simulink model "benchmark_model_2"  (R2021a)
settings: Solver=ode1  StartTime=0.0  StopTime=Tend  FixedStep=0.0001  MaxStep=0.1  MinStep=0.0001  AbsTol=0.01  EnableMultiTasking=on
values from neighbouring files (symbols this model uses):
  A1 = 0.00017774967488    [engine_data.mat]
  A2 = 740220.330082    [engine_data.mat]
  AL = [6 6.5 7 7.5 8 8.5 9 9.5 10 10.5 11 11.5 ... (33 elements, 33x1)]    [engine_data.mat]
  AM0 = 0.02884    [engine_data.mat]
  AREA = 0.00580880481649    [engine_data.mat]
  BORE = 0.086    [engine_data.mat]
  C_EGR = 1.5    [engine_data.mat]
  c_f = 800000    [engine_data.mat]
  c_T = 1    [engine_data.mat]
  CAIR = [0 0 0 0.21 0 0 0.79]    [engine_data.mat]
  cCO = 0    [engine_data.mat]
  cCO2 = 0    [engine_data.mat]
  cH2 = 0    [engine_data.mat]
  cH2O = 0    [engine_data.mat]
  cHC = 0    [engine_data.mat]
  cN2 = 0.79    [engine_data.mat]
  CO = [22.3416398376 20.8398063107 19.3759939408 17.9445472871 16.538827802 15.1528221174 13.7819470707 12.4234138404 11.076283262 9.74128071245 8.42044156849 7.11667724438 ... (33 elements, 33x1)]    [engine_data.mat]
  CO2 = [1.08016197936 1.63070203699 2.20578946805 2.80905596198 3.44329822989 4.11013545224 4.80975559522 5.54078746844 6.30033629562 7.08419123341 7.88717005398 8.70352822078 ... (33 elements, 33x1)]    [engine_data.mat]
  cO2 = 0.21    [engine_data.mat]
  DEN0 = 1.17881164668    [engine_data.mat]
  EGR_dia = 0.02    [engine_data.mat]
  EGR_sk = 0.125663706144    [engine_data.mat]
  EX_AREA = 0.00137444678595    [engine_data.mat]
  EX_M_AR = 0.0258532162804    [engine_data.mat]
  EXO = 40    [engine_data.mat]
  FD0 = 5    [engine_data.mat]
  FOM = [12 11.348 6.233 5 5.449 8.523 5]    [engine_data.mat]
  FR0 = 0    [engine_data.mat]
  FR_C1 = 305.731    [engine_data.mat]
  FR_C2 = 1.70183    [engine_data.mat]
  FR_C3 = 3188.7424    [engine_data.mat]
  FR_C4 = 0.000296028194151    [engine_data.mat]
  FR_C5 = 1.03    [engine_data.mat]
  H2 = [17.3855302766 15.0102176452 12.8820660449 10.9850020715 9.30240027035 7.81790027685 6.51548255669 5.37933989743 4.39378660966 3.5433012035 2.8127075229 2.1874445405 ... (33 elements, 33x1)]    [engine_data.mat]
  H2O = [3.81120036781 5.32559240945 6.64944794012 7.79700886885 8.78142378855 9.61507632366 10.310008356 10.8782622871 11.3320540899 11.6837509075 11.9456809954 12.1298414055 ... (33 elements, 33x1)]    [engine_data.mat]
  HC = [5481.3024964 4476.06435729 3754.34247414 3215.30411383 2799.83726136 2471.30975971 2205.97110777 1987.83348465 1805.78690133 1651.89669698 1520.35918152 1406.8402103 ... (33 elements, 33x1)]    [engine_data.mat]
  INC = 0    [engine_data.mat]
  INO = -40    [engine_data.mat]
  KET = 0.001    [engine_data.mat]
  Kex = 1.28224854645    [engine_data.mat]
  Kh = 0.00462    [engine_data.mat]
  MAS0 = 0.00471524658673    [engine_data.mat]
  MCh = 0.000588883862304    [engine_data.mat]
  MHC = 0.01383448    [engine_data.mat]
  MN2 = 0.028    [engine_data.mat]
  MO2 = 0.032    [engine_data.mat]
  MOLcylT = 0.00157069204711    [engine_data.mat]
  N2 = [54.5020363032 56.4529864816 58.2465252261 59.8999246568 61.4284172656 62.8453054261 64.1621746691 65.3891205654 66.5349581592 67.6074047194 68.6132342687 69.5584035698 ... (33 elements, 33x1)]    [engine_data.mat]
  O2 = [0.331300985803 0.293088680307 0.264743132617 0.242930742419 0.225648917415 0.211629427842 0.200034641439 0.190292592782 0.182002893523 0.174881554044 0.168729672297 0.163420998081 ... (33 elements, 33x1)]    [engine_data.mat]
  PR0 = 101324.72    [engine_data.mat]
  R150 = 157.079632679    [engine_data.mat]
  Rabs = 8.31441    [engine_data.mat]
  SPEC = [4 0.086 0.086 0.043 0.14665 14 1 0.1 0 0.5 0.005 0 ... (19 elements, 19x1)]    [engine_data.mat]
  TBORE = 0.055    [engine_data.mat]
  Tend = 120    [engine_data.mat]
  Th_HC = 0.1    [engine_data.mat]
  Th_knock = 0.401961937891    [engine_data.mat]
  THEX = [0 1 2 3 4 5 6 7 8 9 10 11 ... (721 elements, 1x721)]    [engine_data.mat]
  THIN = [0 1 2 3 4 5 6 7 8 9 10 11 ... (721 elements, 1x721)]    [engine_data.mat]
  TM0 = 298.15    [engine_data.mat]
  Tstart = 5    [engine_data.mat]
  TW0 = 353.15    [engine_data.mat]
  V_EX = 0.0001    [engine_data.mat]
  VAREX = [0 0 0 0 0 0 0 0 0 0 0 0 ... (721 elements, 1x721)]    [engine_data.mat]
  VARIN = [0 0 0 0 0 0 0 0 0 0 0 0 ... (721 elements, 1x721)]    [engine_data.mat]
  VH = 0.000499557214218    [engine_data.mat]
  VT = 3.84274780168e-05    [engine_data.mat]
  WOM = [0.01383448 0.04401 0.02801 0.032 0.002016 0.018016 0.028]    [engine_data.mat]
  y = 1.81    [engine_data.mat]
undefined symbols (not defined in the file or in its folder): DiscIntNeverNeededParam
libraries: pid_lib x3
(part 7 of 7)

== matlab function benchmark_model_2/ENGINE/engine_s/cylinders/cyl2/cyl/frame/ratio_burnt1/murnt_ratio/Embedded MATLAB Function ==
  data: u input; q output; Web input; Q output
function [q,Q]  = func_webC_s(u,Web)
% made by Alex on January 28th, 2010
%   y: burnt ratio
%   u: crank angle that takes 0 at the compression TDC
% Web: parameters
%
WebA = Web(1);
WebM = Web(2);
WebT = Web(3);
WebS = Web(4);
WWebs = pi-WebS;

uu = mod(u,4*pi)-WWebs;
if (uu>0)   
    q = 1.0/WebT*(WebM+1.0)*WebA*(uu/WebT)^WebM*...
          exp(-WebA*(uu/WebT)^(WebM+1.0));
    Q = 1-exp(-WebA*(uu/WebT)^(WebM+1.0));
else
    q = 0;
    Q = 0;
end

== matlab function benchmark_model_2/ENGINE/engine_s/ex_chamber/cal_flow ==
  data: area input; fen output; inlet input; c_in input; outlet input; c_out input; fml output; WOM input
function [fen,fml] = func_nozzle(area,inlet,c_in,outlet,c_out,WOM) 
% made by Alex on February 3rd, 2010
% This program calculates the flow rate through the nozzle 
% under the assamption that the mass, the energy and the mometum
% are conserved between the inlet and the outlet flows.
%
% The inlet and the outlet are connected with the sign convention 
% of the calculated flow. The sign of the flow from th einlet and 
% the outlet is positive.
%
% inlet(1):pressure 
% inlet(2):density
% inlet(3):weight of molecule
% inlet(4):degree of freedom
% outlet(1):pressure 
% outlet(2):density
% outlet(3):weight of molecule
% outlet(4):degree of freedom

y = zeros(8,1); % modified 

du = inlet(1);
if du<0
    du=0;
end
pu = inlet(2);
mu = inlet(3);
fu = inlet(4);
dd = outlet(1);
pd = outlet(2);
md = outlet(3);
fd = outlet(4);
AR = area;

if (pu >= pd)
    rp = pd/pu;
    k = (fu + 2.0)/fu;
    crp = 1.0/(k + 1.0);
    A = AR*sqrt((k + 1.0)/(2.0*k)*pu*du);
    B = sqrt((k/(k + 1.0))^2 - (0.99 - 1.0/(k + 1.0))^2);
    C = -(0.99 - 1.0/(k + 1.0))/B;
    a = (C*0.01 - B)/(2.0*0.01^3);
    c = C - 3.0*a*0.01^2;
    if (rp >= 0.99)
      fms = A*(a*(1.0 - rp)^3 + c*(1.0 - rp));
    else
      if (rp >= crp)
        R = (k/(k + 1.0))^2 - (rp - 1.0/(k + 1.0))^2;
        if (R < 0)
          R = 0;
        end
        fms = A*sqrt(R);
      else
        fms = A*k/(k + 1.0);
      end
    end
    fen = fms*(fu + 2.0)/2.0*pu/du;
    Ma = WOM'*c_in;
    fml = c_in*fms/Ma;
  else
    rp = pu/pd;
    k = (fd + 2.0)/fd;
    crp = 1.0/(k + 1.0);
    A = AR*sqrt((k + 1.0)/(2.0*k)*pd*dd);
    B = sqrt((k/(k + 1.0))^2 - (0.99 - 1.0/(k + 1.0))^2);
    C = (0.99 - 1.0/(k + 1.0))/B;
    a = (C*0.01 - B)/(2.0*0.01^3);
    c = C - 3.0*a*0.01^2;
    if (rp >= 0.99)
      fms = -A*(a*(1.0 - rp)^3 + c*(1.0 - rp));
    else
      if (rp >= crp)
        R = (k/(k + 1.0))^2 - (rp - 1.0/(k + 1.0))^2;
        if (R < 0)
          R = 0;
        end
        fms = -A*sqrt(R);
      else
        fms = -A*k/(k + 1.0);
      end
    end
    fen = fms*(fd + 2.0)/2.0*pd/dd;
    Ma = WOM'*c_out;
    fml = c_out*fms/Ma;
end
if isnan(fen)
       fen=0;
end

== stateflow chart benchmark_model_2/ENGINE/engine_s/cylinders/cyl2/cyl/unburnt_gass/init&trig/qChart ==
  state A/
    exit:
    sl_out1=sl_in1;
    sl_out2=sl_in2;
    sl_out3=sl_in3;
    sl_out4=sl_in4;
    sl_out5=sl_in5;
    sl_out6=sl_in6;
    sl_out7=sl_in7;
  (default) -> A : {sl_out1=sl_in1;
      |  sl_out2=sl_in2;
      |  sl_out3=sl_in3;
      |  sl_out4=sl_in4;
      |  sl_out5=sl_in5;
      |  sl_out6=sl_in6;
      |  sl_out7=sl_in7;
      | }
  A -> A : event
  data: sl_in1 input; sl_out1 output double =NHC; sl_in2 input; sl_in3 input; sl_in4 input; sl_in5 input; sl_in6 input; sl_in7 input; sl_out2 output double =NCO2; sl_out3 output double =NCO; sl_out4 output double =NO2; sl_out5 output double =NH2; sl_out6 output double =NH2O; sl_out7 output double =NN2
  events: event input RISING_EDGE_EVENT

== matlab function benchmark_model_2/ENGINE/engine_s/cylinders/cyl2/ex_valve/cal_flow ==
  data: area input; fen output; inlet input; c_in input; outlet input; c_out input; fml output; WOM input
function [fen,fml] = func_nozzle(area,inlet,c_in,outlet,c_out,WOM) 
% made by Alex on February 3rd, 2010
% This program calculates the flow rate through the nozzle 
% under the assamption that the mass, the energy and the mometum
% are conserved between the inlet and the outlet flows.
%
% The inlet and the outlet are connected with the sign convention 
% of the calculated flow. The sign of the flow from th einlet and 
% the outlet is positive.
%
% inlet(1):pressure 
% inlet(2):density
% inlet(3):weight of molecule
% inlet(4):degree of freedom
% outlet(1):pressure 
% outlet(2):density
% outlet(3):weight of molecule
% outlet(4):degree of freedom

y = zeros(8,1); % modified 

du = inlet(1);
pu = inlet(2);
if pu<0
    pu=0;
end
mu = inlet(3);
fu = inlet(4);
dd = outlet(1);
if dd<0
    dd=0;
end
pd = outlet(2);
md = outlet(3);
fd = outlet(4);
AR = area;

if (pu >= pd)
    rp = pd/pu;
    k = (fu + 2.0)/fu;
    crp = 1.0/(k + 1.0);
    A = AR*sqrt((k + 1.0)/(2.0*k)*pu*du);
    B = sqrt((k/(k + 1.0))^2 - (0.99 - 1.0/(k + 1.0))^2);
    C = -(0.99 - 1.0/(k + 1.0))/B;
    a = (C*0.01 - B)/(2.0*0.01^3);
    c = C - 3.0*a*0.01^2;
    if (rp >= 0.99)
      fms = A*(a*(1.0 - rp)^3 + c*(1.0 - rp));
    else
      if (rp >= crp)
        R = (k/(k + 1.0))^2 - (rp - 1.0/(k + 1.0))^2;
        if (R < 0)
          R = 0;
        end
        fms = A*sqrt(R);
      else
        fms = A*k/(k + 1.0);
      end
    end
    fen = fms*(fu + 2.0)/2.0*pu/du;
    Ma = WOM'*c_in;
    fml = c_in*fms/Ma;
  else
    rp = pu/pd;
    k = (fd + 2.0)/fd;
    crp = 1.0/(k + 1.0);
    A = AR*sqrt((k + 1.0)/(2.0*k)*pd*dd);
    B = sqrt((k/(k + 1.0))^2 - (0.99 - 1.0/(k + 1.0))^2);
    C = (0.99 - 1.0/(k + 1.0))/B;
    a = (C*0.01 - B)/(2.0*0.01^3);
    c = C - 3.0*a*0.01^2;
    if (rp >= 0.99)
      fms = -A*(a*(1.0 - rp)^3 + c*(1.0 - rp));
    else
      if (rp >= crp)
        R = (k/(k + 1.0))^2 - (rp - 1.0/(k + 1.0))^2;
        if (R < 0)
          R = 0;
        end
        fms = -A*sqrt(R);
      else
        fms = -A*k/(k + 1.0);
      end
    end
    fen = fms*(fd + 2.0)/2.0*pd/dd;
    Ma = WOM'*c_out;
    fml = c_out*fms/Ma;
end
if isnan(fen)
       fen=0;
end

== matlab function benchmark_model_2/ENGINE/engine_s/cylinders/cyl2/in_valve/cal_flow ==
  data: area input; fen output; inlet input; c_in input; outlet input; c_out input; fml output; fms output; WOM input
function [fen,fml,fms] = func_nozzle(area,inlet,c_in,outlet,c_out,WOM) 
% made by Alex on February 3rd, 2010
% This program calculates the flow rate through the nozzle 
% under the assamption that the mass, the energy and the mometum
% are conserved between the inlet and the outlet flows.
%
% The inlet and the outlet are connected with the sign convention 
% of the calculated flow. The sign of the flow from th einlet and 
% the outlet is positive.
%
% inlet(1):pressure 
% inlet(2):density
% inlet(3):weight of molecule
% inlet(4):degree of freedom
% outlet(1):pressure 
% outlet(2):density
% outlet(3):weight of molecule
% outlet(4):degree of freedom

y = zeros(8,1); % modified 
du = inlet(1);
if du<0
    du=0;
end
pu = inlet(2);
mu = inlet(3);
fu = inlet(4);
dd = outlet(1);
if dd<0
    dd=1e-9;
end
pd = outlet(2);
md = outlet(3);
fd = outlet(4);
AR = area;

if (pu >= pd)
    rp = pd/pu;
    k = (fu + 2.0)/fu;
    crp = 1.0/(k + 1.0);
    A = AR*sqrt((k + 1.0)/(2.0*k)*pu*du);
    B = sqrt((k/(k + 1.0))^2 - (0.99 - 1.0/(k + 1.0))^2);
    C = -(0.99 - 1.0/(k + 1.0))/B;
    a = (C*0.01 - B)/(2.0*0.01^3);
    c = C - 3.0*a*0.01^2;
    if (rp >= 0.99)
      fms = A*(a*(1.0 - rp)^3 + c*(1.0 - rp));
    else
      if (rp >= crp)
        R = (k/(k + 1.0))^2 - (rp - 1.0/(k + 1.0))^2;
        if (R < 0)
          R = 0;
        end
        fms = A*sqrt(R);
      else
        fms = A*k/(k + 1.0);
      end
    end
    fen = fms*(fu + 2.0)/2.0*pu/du;
    Ma = WOM'*c_in;
    fml = c_in*fms/Ma;
  else
    rp = pu/pd;
    k = (fd + 2.0)/fd;
    crp = 1.0/(k + 1.0);
    A = AR*sqrt((k + 1.0)/(2.0*k)*pd*dd);
    B = sqrt((k/(k + 1.0))^2 - (0.99 - 1.0/(k + 1.0))^2);
    C = (0.99 - 1.0/(k + 1.0))/B;
    a = (C*0.01 - B)/(2.0*0.01^3);
    c = C - 3.0*a*0.01^2;
    if (rp >= 0.99)
      fms = -A*(a*(1.0 - rp)^3 + c*(1.0 - rp));
    else
      if (rp >= crp)
        R = (k/(k + 1.0))^2 - (rp - 1.0/(k + 1.0))^2;
        if (R < 0)
          R = 0;
        end
        fms = -A*sqrt(R);
      else
        fms = -A*k/(k + 1.0);
      end
    end
    fen = fms*(fd + 2.0)/2.0*pd/dd;
    Ma = WOM'*c_out;
    fml = c_out*fms/Ma;
end
 if isnan(fen)
       fen=0;
end
